simulink model "UpdownCounter_using_Stateflow"  (R2023b)
settings: Solver=FixedStepDiscrete  StartTime=0.0  StopTime=1  FixedStep=0.01  RelTol=1e-3
settings Model: Creator=Pranav  LastModifiedBy=Pranav

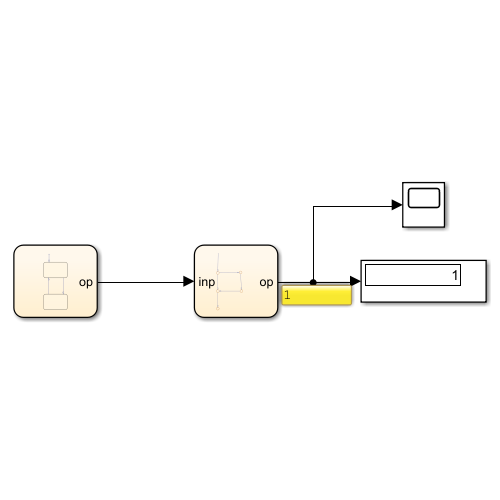
[thumbnail: Simulink's stored preview of the top-level diagram]
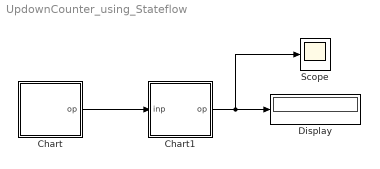
== system UpdownCounter_using_Stateflow ==
  Chart : Stateflow chart  TreatAsAtomicUnit=on
  Chart1 : Stateflow chart  TreatAsAtomicUnit=on
  Display : Display
  Scope : Scope
  wires:
  Chart/1(op) -> Chart1/1(inp)
  Chart1/1(op) -> Scope/1, Display/1

== stateflow chart UpdownCounter_using_Stateflow/Chart1 ==
  (default) -> (junction 1)
  (junction 1) -> (junction 3) [order 1] : [inp==1&&i<=10]
  (junction 3) -> (junction 5) : {i = i + 1;
      | op=i;}
  (junction 1) -> (junction 7) [order 2] : {
      | i = i - 1;
      | op=i;}
  (junction 5) -> (junction 7)
  (junction 7) -> (junction 12)
  data: inp input; i local =0; op output

== stateflow chart UpdownCounter_using_Stateflow/Chart ==
  state Control
    op=1;
  state Control1
    op=0;
  (default) -> Control
  Control1 -> Control : after(0.10,sec)
  Control -> Control1 : after(0.10,sec)
  data: op output
